simulink model "Tets"  (R2020b)
settings: Solver=FixedStepAuto  StartTime=0.0  StopTime=inf  FixedStep=0.02  RelTol=1e-3
settings Model: Creator=GW00216231  LastModifiedBy=GW00216231

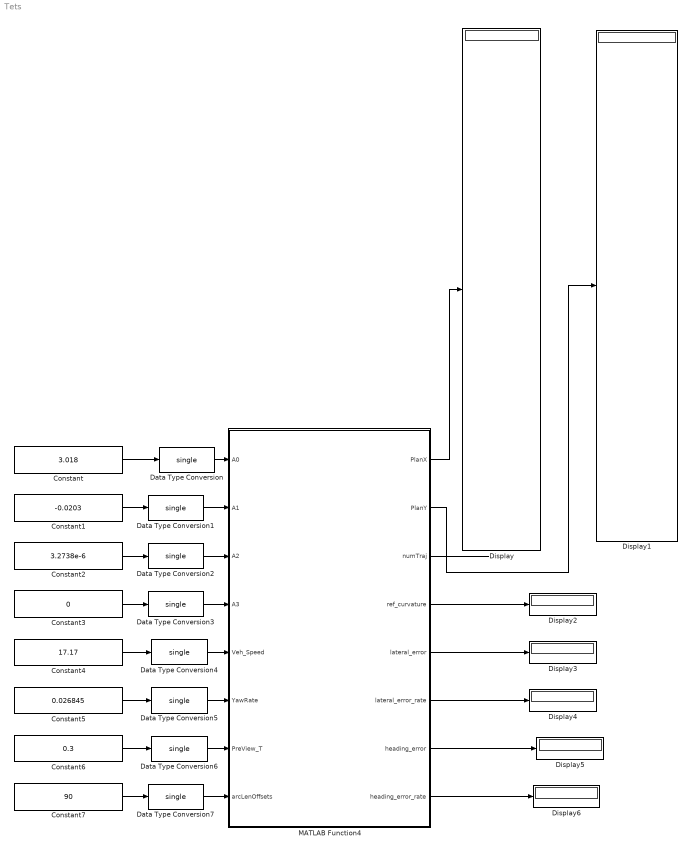
== system Tets ==
  Constant : Constant  Value=3.018
  Constant1 : Constant  Value=-0.0203
  Constant2 : Constant  Value=3.2738e-6
  Constant3 : Constant  Value=0
  Constant4 : Constant  Value=17.17
  Constant5 : Constant  Value=0.026845
  Constant6 : Constant  Value=0.3
  Constant7 : Constant  Value=90
  Data Type Conversion{,1..7} (8 alike) : DataTypeConversion  OutDataTypeStr=single
  Display{,1..6} (7 alike) : Display
  MATLAB Function4 : MATLAB Function  TreatAsAtomicUnit=on
  wires:
  Constant4/1 -> Data Type Conversion4/1
  Constant3/1 -> Data Type Conversion3/1
  Constant2/1 -> Data Type Conversion2/1
  Constant1/1 -> Data Type Conversion1/1
  Constant/1 -> Data Type Conversion/1
  Constant5/1 -> Data Type Conversion5/1
  Constant6/1 -> Data Type Conversion6/1
  Constant7/1 -> Data Type Conversion7/1
  MATLAB Function4/1(PlanX) -> Display/1
  MATLAB Function4/2(PlanY) -> Display1/1
  MATLAB Function4/3(numTraj) -> ?
  MATLAB Function4/4(ref_curvature) -> Display2/1
  MATLAB Function4/5(lateral_error) -> Display3/1
  MATLAB Function4/6(lateral_error_rate) -> Display4/1
  MATLAB Function4/7(heading_error) -> Display5/1
  MATLAB Function4/8(heading_error_rate) -> Display6/1
  Data Type Conversion/1 -> MATLAB Function4/1(A0)
  Data Type Conversion1/1 -> MATLAB Function4/2(A1)
  Data Type Conversion2/1 -> MATLAB Function4/3(A2)
  Data Type Conversion3/1 -> MATLAB Function4/4(A3)
  Data Type Conversion4/1 -> MATLAB Function4/5(Veh_Speed)
  Data Type Conversion5/1 -> MATLAB Function4/6(YawRate)
  Data Type Conversion6/1 -> MATLAB Function4/7(PreView_T)
  Data Type Conversion7/1 -> MATLAB Function4/8(arcLenOffsets)

== matlab function Tets/MATLAB Function4 ==
  data: A0 input; A1 input; A2 input; A3 input; Veh_Speed input size=1; YawRate input size=1; PreView_T input size=1; PlanX output; PlanY output; numTraj output size=1; ref_curvature output; arcLenOffsets input size=1; lateral_error output size=1; lateral_error_rate output size=1; heading_error output size=1; heading_error_rate output size=1
function [PlanX,PlanY,numTraj,ref_curvature,lateral_error,lateral_error_rate,heading_error,heading_error_rate]= fcn(A0,A1,A2,A3,Veh_Speed,YawRate,PreView_T,arcLenOffsets)
% 参考线离散化
rx1 = [single(0):single(1):single(9)];
rx2 = [single(10):20:150];
rx = cat(2,rx1,rx2);
ry = single((-1)).*(A0 + A1.* rx + A2.* (rx.^2) + A3.* (rx.^3));
waypoints = [ry',rx'];
referencePath = FrenentReferencePath(waypoints,20);
pathStart = referencePath.interpolate(0);% 求起始点处车辆状态 [x, y,theta, kappa, dkappa, s]
initialState=[0 -A0 pathStart(1,3)];

Frenet_traj_obj = TrajectoryGeneratorFrenet(referencePath);
% arcLenOffsets = single(60);
FtNumTarpoints = single(40);
GtNumTarpoints = single(40);
[frenetTrajectory,globalTrajectory,numTraj] = Frenet_traj_obj.FrenetTrajectory_Lateral(initialState,arcLenOffsets,0,FtNumTarpoints,GtNumTarpoints);
[globalTrajectory] = EvaluateTrajectory_Lateral(frenetTrajectory,globalTrajectory, 1,1);
% [s,d]→[x, y, theta, kappa, dkappa]
FB = single(zeros(40,1));
PlanY = single(zeros(40,1));
PlanX= globalTrajectory(1).Trajectory(1:40,2);
PlanY= globalTrajectory(1).Trajectory(1:40,1);
[matrix_state,ref_curvature] = Calc_State_Error(Veh_Speed,YawRate,globalTrajectory,PreView_T);
% lateral_error = single(zeros(1,1));lateral_error_rate = single(zeros(1,1));heading_error = single(zeros(1,1));heading_error_rate = single(zeros(1,1));
lateral_error = matrix_state(1,1);
lateral_error_rate = matrix_state(2,1);
heading_error = matrix_state(3,1);
heading_error_rate = matrix_state(4,1);
end
